simulink model "simtcs_V1"  (R2018a)
settings: Solver=VariableStepAuto  StartTime=0.0  StopTime=10.0  RelTol=1e-3
values from neighbouring files (symbols this model uses):
  alfa = rw/((Jm*n)+(Jw/n))    (= 1.25820007017)    [TCS.m]
  Fz = m*9.81    (= 1962)    [TCS.m]
  k1 = K(1,1)    [TCS.m]
  K1 = 6.5    [TCS.m]
  k2 = K(1,2)    [TCS.m]
  K2 = 1.54    [TCS.m]
  k3 = K(1,3)    [TCS.m]
  K3 = -1    [TCS.m]
  K4 = -4    [TCS.m]
  Km = 2.0    (= 2)    [TCS.m]
  m = 200    [TCS.m]
  n = 6.267    [TCS.m]
  rw = 0.225    [TCS.m]
  tau_m = 0.007    [TCS.m]
settings Model: Creator=aoki-soya  LastModifiedBy=aoki-soya

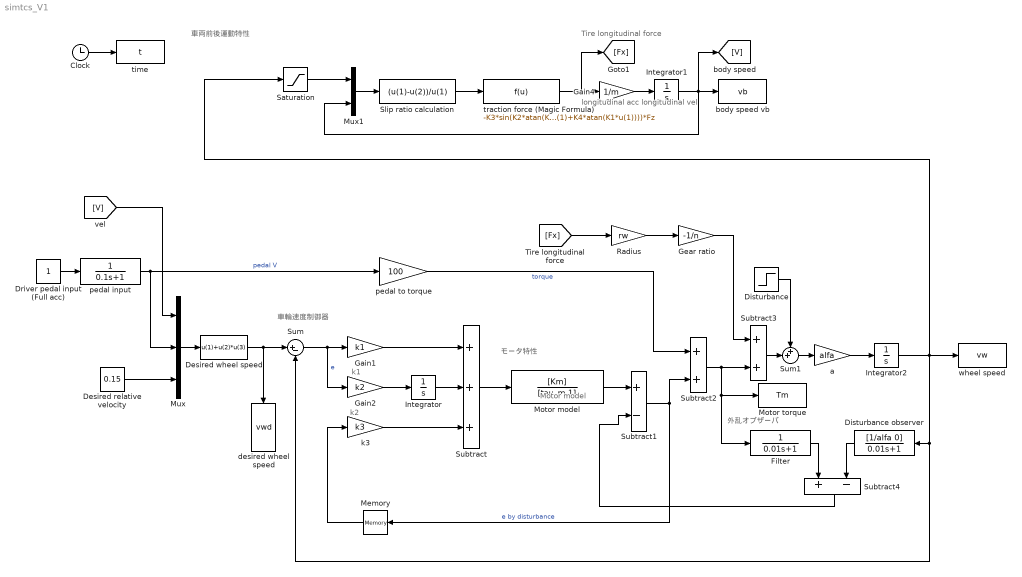
== system simtcs_V1 ==
  note: 外乱オブザーバ
  note: モータ特性
  note: 車輪速度制御器
  note: 車両前後運動特性
  note: longitudinal vel
  note: longitudinal acc
  note: Tire longitudinal force
  note: Motor model
  note: k2
  note: k1
  Clock : Clock
  Desired relative velocity : Constant  Value=0.15
  Desired wheel speed : Fcn  Expr=u(1)+u(2)*u(3)
  Disturbance : Step  After=10  SampleTime=0
  Disturbance observer : TransferFcn  Numerator=[1/alfa 0]  Denominator=[0.01 1]
  Driver pedal input (Full acc) : Constant
  Filter : TransferFcn  Denominator=[0.01 1]
  Gain1 : Gain  Gain=k1
  Gain2 : Gain  Gain=k2
  Gain4 : Gain  Gain=1/m
  Gear ratio : Gain  Gain=-1/n
  Integrator : Integrator  LimitOutput=on  LowerSaturationLimit=0
  Integrator1 : Integrator
  Integrator2 : Integrator  LimitOutput=on  LowerSaturationLimit=0
  Memory : Memory
  Motor model : TransferFcn  Numerator=[Km]  Denominator=[tau_m 1]
  Motor torque : ToWorkspace  VariableName=Tm  SaveFormat=Timeseries  SampleTime=-1
  Mux : Mux  Inputs=3
  Mux1 : Mux  Inputs=2
  Radius : Gain  Gain=rw
  Saturation : Saturate  UpperLimit=inf  LowerLimit=0.001
  Slip ratio calculation : Fcn  Expr=(u(1)-u(2))/u(1)
  Subtract : Sum  Inputs=+++
  Subtract1 : Sum  Inputs=+-
  Subtract2 : Sum
  Subtract3 : Sum
  Subtract4 : Sum  Inputs=+-
  Sum : Sum  Inputs=|+-
  Sum1 : Sum  Inputs=++|
  a : Gain  Gain=alfa
  body speed vb : ToWorkspace  VariableName=vb  SaveFormat=Timeseries  SampleTime=-1
  desired wheel speed : ToWorkspace  VariableName=vwd  SaveFormat=Timeseries  SampleTime=-1
  "k3 " : Gain  Gain=k3
  pedal input : TransferFcn  Denominator=[0.1 1]
  pedal to torque : Gain  Gain=100
  time : ToWorkspace  VariableName=t  SaveFormat=Timeseries  SampleTime=-1
  traction force (Magic Formula) : Fcn  Expr=-K3*sin(K2*atan(K1*(1-K4)*u(1)+K4*atan(K1*u(1))))*Fz
  wheel speed : ToWorkspace  VariableName=vw  SaveFormat=Timeseries  SampleTime=-1
  wires:
  Clock/1 -> time/1
  Driver pedal input (Full acc)/1 -> pedal input/1
  pedal input/1 -> pedal to torque/1, Mux/2  "pedal V"
  [V] -> Mux/1
  Desired relative velocity/1 -> Mux/3
  Mux/1 -> Desired wheel speed/1
  Desired wheel speed/1 -> Sum/1, desired wheel speed/1
  Sum/1 -> Gain2/1, Gain1/1  "e"
  Gain2/1 -> Integrator/1
  Gain1/1 -> Subtract/1
  Integrator/1 -> Subtract/2
  "k3 "/1 -> Subtract/3
  Subtract/1 -> Motor model/1
  Motor model/1 -> Subtract1/1
  Subtract1/1 -> Memory/1, Subtract2/2  "e by disturbance"
  pedal to torque/1 -> Subtract2/1  "torque"
  Memory/1 -> "k3 "/1
  traction force (Magic Formula)/1 -> [Fx], Gain4/1
  Slip ratio calculation/1 -> traction force (Magic Formula)/1
  Gain4/1 -> Integrator1/1
  Integrator1/1 -> Mux1/2, [V], body speed vb/1
  Mux1/1 -> Slip ratio calculation/1
  [Fx] -> Radius/1
  Radius/1 -> Gear ratio/1
  Gear ratio/1 -> Subtract3/1
  a/1 -> Integrator2/1
  Saturation/1 -> Mux1/1
  Subtract2/1 -> Filter/1, Motor torque/1, Subtract3/2
  Filter/1 -> Subtract4/1
  Disturbance observer/1 -> Subtract4/2
  Subtract4/1 -> Subtract1/2
  Integrator2/1 -> Sum/2, Disturbance observer/1, wheel speed/1, Saturation/1
  Subtract3/1 -> Sum1/2
  Disturbance/1 -> Sum1/1
  Sum1/1 -> a/1
